simulink model "NewModel"  (R2024b)
settings: Solver=FixedStepDiscrete  StartTime=0.0  StopTime=6.0  FixedStep=2.0  RelTol=1e-3
settings Model: Creator=saijaz  LastModifiedBy=saijaz

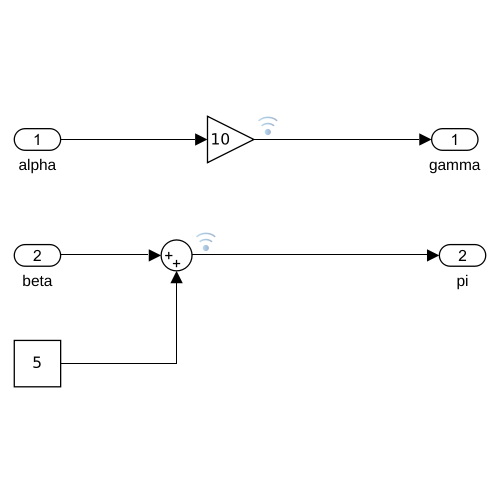
[thumbnail: Simulink's stored preview of the top-level diagram]
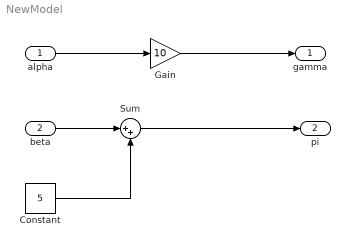
== system NewModel ==
  alpha : Inport  OutDataTypeStr=single
  beta : Inport  Port=2  OutDataTypeStr=uint8
  Constant : Constant  Value=5  OutDataTypeStr=uint8
  Gain : Gain  Gain=10
  Sum : Sum  Inputs=|++
  gamma : Outport  OutDataTypeStr=single
  pi : Outport  Port=2  OutDataTypeStr=uint8
  wires:
  alpha/1 -> Gain/1
  Gain/1 -> gamma/1
  beta/1 -> Sum/1
  Sum/1 -> pi/1
  Constant/1 -> Sum/2
